simulink model "robot_3DoF_model"  (R2023a)
settings: Solver=FixedStepDiscrete  StartTime=0.0  StopTime=Inf  FixedStep=Ts_integration  RelTol=1e-3  EnableMultiTasking=on
model workspace (MAT data in the model file):
  Board = Simulink.Parameter
  Board.Value = [0.4  0.4; 0.2  0.6; 0  0.4]
  Board.DataType = 'double'
  Board.Complexity = 'real'
  Board.Dimensions = [3 2]
  BoardStiffness = Simulink.Parameter
  BoardStiffness.Value = [1000  0  0; 0  0  0; 0  0  0]
  BoardStiffness.DataType = 'auto'
  BoardStiffness.Complexity = 'real'
  BoardStiffness.Dimensions = [3 3]
  HC_KfD = Simulink.Parameter
  HC_KfD.Value = [0.1  0  0; 0  0  0; 0  0  0]
  HC_KfD.DataType = 'double'
  HC_KfD.Complexity = 'real'
  HC_KfD.Dimensions = [3 3]
  HC_KfI = Simulink.Parameter
  HC_KfI.Value = [1  0  0; 0  0  0; 0  0  0]
  HC_KfI.DataType = 'double'
  HC_KfI.Complexity = 'real'
  HC_KfI.Dimensions = [3 3]
  HC_KfP = Simulink.Parameter
  HC_KfP.Value = [0.05  0  0; 0  0  0; 0  0  0]
  HC_KfP.DataType = 'double'
  HC_KfP.Complexity = 'real'
  HC_KfP.Dimensions = [3 3]
  HC_KpD = Simulink.Parameter
  HC_KpD.Value = [15  0  0; 0  15  0; 0  0  20]
  HC_KpD.DataType = 'double'
  HC_KpD.Complexity = 'real'
  HC_KpD.Dimensions = [3 3]
  HC_KpI = Simulink.Parameter
  HC_KpI.Value = [0.5  0  0; 0  0.5  0; 0  0  10]
  HC_KpI.DataType = 'double'
  HC_KpI.Complexity = 'real'
  HC_KpI.Dimensions = [3 3]
  HC_KpP = Simulink.Parameter
  HC_KpP.Value = [25  0  0; 0  25  0; 0  0  600]
  HC_KpP.DataType = 'double'
  HC_KpP.Complexity = 'real'
  HC_KpP.Dimensions = [3 3]
  HC_Selection = Simulink.Parameter
  HC_Selection.Value = [0  0  0; 0  1  0; 0  0  1]
  HC_Selection.DataType = 'double'
  HC_Selection.Complexity = 'real'
  HC_Selection.Dimensions = [3 3]
  HC_tau0 = Simulink.Parameter
  HC_tau0.Value = [0; 0; 12.3985]
  HC_tau0.DataType = 'double'
  HC_tau0.Complexity = 'real'
  HC_tau0.Dimensions = [3 1]
  SM_gamma = Simulink.Parameter
  SM_gamma.Value = 0.001
  SM_gamma.DataType = 'auto'
  SM_gamma.Complexity = 'real'
  SM_gamma.Dimensions = [1 1]
  SM_lambda = Simulink.Parameter
  SM_lambda.Value = 2
  SM_lambda.DataType = 'auto'
  SM_lambda.Complexity = 'real'
  SM_lambda.Dimensions = [1 1]
  SM_rho = Simulink.Parameter
  SM_rho.Value = 10
  SM_rho.DataType = 'auto'
  SM_rho.Complexity = 'real'
  SM_rho.Dimensions = [1 1]
  SM_slidingGain = Simulink.Parameter
  SM_slidingGain.Value = [0  0  0; 0  0  0; 0  0  0]
  SM_slidingGain.DataType = 'auto'
  SM_slidingGain.Complexity = 'real'
  SM_slidingGain.Dimensions = [3 3]
  SM_widthInverse = Simulink.Parameter
  SM_widthInverse.Value = [100  0  0; 0  100  0; 0  0  100]
  SM_widthInverse.DataType = 'auto'
  SM_widthInverse.Complexity = 'real'
  SM_widthInverse.Dimensions = [3 3]
  Ts_control = Simulink.Parameter
  Ts_control.Value = 0.01
  Ts_control.DataType = 'double'
  Ts_control.Complexity = 'real'
  Ts_control.Dimensions = [1 1]
  Ts_integration = Simulink.Parameter
  Ts_integration.Value = 0.001
  Ts_integration.DataType = 'double'
  Ts_integration.Complexity = 'real'
  Ts_integration.Dimensions = [1 1]
  q_initial = Simulink.Parameter
  q_initial.Value = [2.00142; -1.6713; -0.21737; 0; 0; 0]
  q_initial.DataType = 'double'
  q_initial.Complexity = 'real'
  q_initial.Dimensions = [6 1]
  q_res1 = Simulink.Parameter
  q_res1.Value = 628318
  q_res1.DataType = 'auto'
  q_res1.Complexity = 'real'
  q_res1.Dimensions = [1 1]
  q_res2 = Simulink.Parameter
  q_res2.Value = 628318
  q_res2.DataType = 'auto'
  q_res2.Complexity = 'real'
  q_res2.Dimensions = [1 1]
  q_res3 = Simulink.Parameter
  q_res3.Value = 628318
  q_res3.DataType = 'auto'
  q_res3.Complexity = 'real'
  q_res3.Dimensions = [1 1]
libraries: dspinverses x1
settings Model: Creator=devans  LastModifiedBy=admin
settings SolverCC: AlgebraicLoopSolver=TrustRegion
settings DataIOCC: SaveFormat=Array  SignalLoggingSaveFormat=ModelDataLogs  SaveOutput=off  SaveTime=off  ReturnWorkspaceOutputs=off  SignalLoggingName=sigsOut
settings OptimizationCC: ExpressionDepthLimit=2147483647  LifeSpan=inf
settings DebuggingCC: SaveWithParameterizedLinksMsg=none  UnderspecifiedInitializationDetection=Classic  MergeDetectMultiDrivingBlocksExec=none  SignalResolutionControl=TryResolveAllWithWarning  MultiTaskDSMMsg=warning  MultiTaskCondExecSysMsg=none  UnconnectedInputMsg=warning  UnconnectedOutputMsg=warning  UnconnectedLineMsg=warning  StateNameClashWarn=warning  SFUnexpectedBacktrackingDiag=warning  SFNoUnconditionalDefaultTransitionDiag=warning  SFExecutionAtInitializationDiag=none  ArithmeticOperatorsInVariantConditions=warning
settings HardwareCC: ProdBitPerPointer=32  ProdBitPerSizeT=32  ProdBitPerPtrDiffT=32  ProdLargestAtomicFloat=None  ProdIntDivRoundTo=Undefined  ProdEndianess=Unspecified  ProdWordSize=32  ProdHWDeviceType=32-bit Generic  TargetBitPerPointer=64  TargetBitPerSizeT=64  TargetBitPerPtrDiffT=64  TargetLongLongMode=on  TargetIntDivRoundTo=Zero  TargetEndianess=LittleEndian  TargetWordSize=64  TargetHWDeviceType=MATLAB Host  ProdEqTarget=off
settings ModelReferenceCC: PropagateSignalLabelsOutOfModel=off
settings SFSimCC: SimUseLocalCustomCode=off  CustomCodeUndefinedFunction=UseInterfaceOnly
settings RTWCC: RTWUseLocalCustomCode=off
settings CodeAppCC: StateflowObjectComments=on
settings GRTTargetCC: TargetLangStandard=C89/C90 (ANSI)  CombineOutputUpdateFcns=off  GRTInterface=on
settings ConfigComp: CovMetricSettings=dw  CovSaveCumulativeToWorkspaceVar=on  CovSaveSingleToWorkspaceVar=on  CovExternalEMLEnable=off

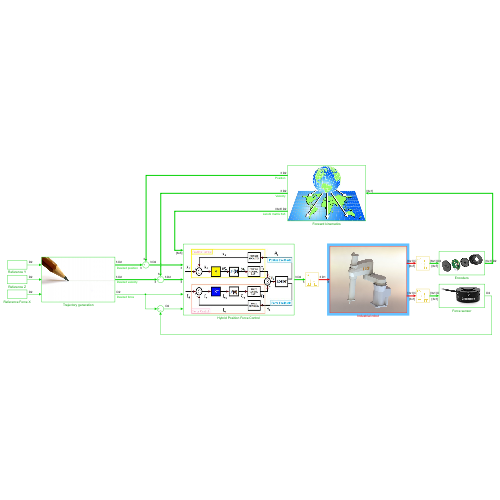
[thumbnail: Simulink's stored preview of the top-level diagram]
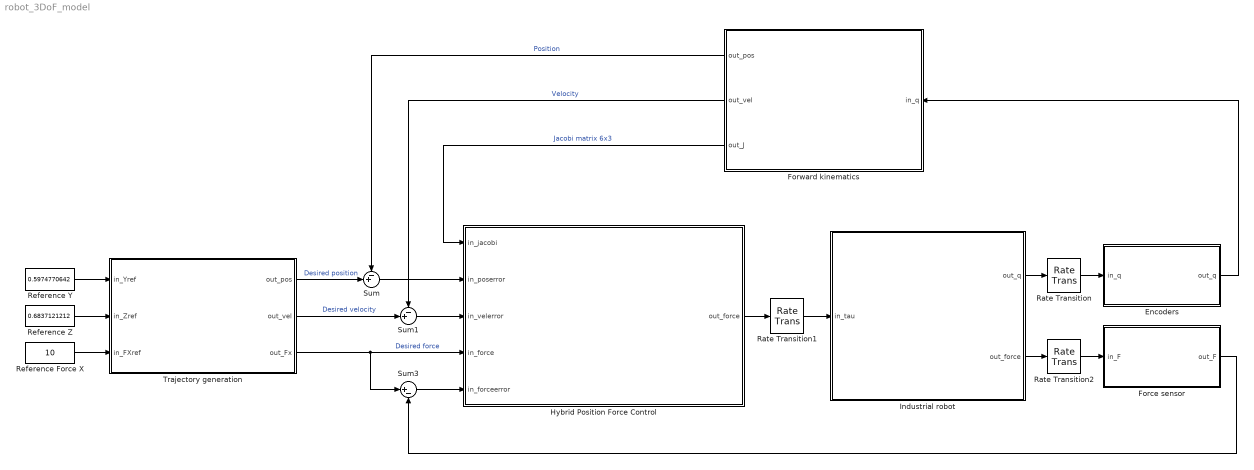
== system robot_3DoF_model ==
  Encoders : Subsystem
      mask Display: image('./Media/MR-Encoder.jpg');
  Force sensor : Subsystem
      mask Display: image('./Media/forcesensor.jpg');
  Forward kinematics : Subsystem
      mask Display: image('./Media/inverse.jpg');
  Hybrid Position Force Control : Subsystem
      mask Display: image('./Media/hybridcontrol.jpg');
  Industrial robot : Subsystem
      mask Display: image('./Media/3DoFrobot.jpg');
  Rate Transition : RateTransition  InitialCondition=q_initial  OutPortSampleTime=Ts_control
  Rate Transition1 : RateTransition  InitialCondition=[0;0;0]  OutPortSampleTime=Ts_integration
  Rate Transition2 : RateTransition  InitialCondition=[0;0;0]  OutPortSampleTime=Ts_control
  Reference Force X : Constant  Value=10  OutMin=5  OutMax=20  SampleTime=Ts_control
  Reference Y : Constant  Value=0.5974770642  OutMin=0  OutMax=1  SampleTime=Ts_control
  Reference Z : Constant  Value=0.6837121212  OutMin=0  OutMax=1  SampleTime=Ts_control
  Sum : Sum  Inputs=-+|
  Sum1 : Sum  Inputs=-+|
  Sum3 : Sum  Inputs=|+-
  Trajectory generation : Subsystem
      mask Display: image('./Media/draw-the-line.jpg');
  wires:
  Industrial robot/1(out_q) -> Rate Transition/1
  Rate Transition/1 -> Encoders/1(in_q)
  Encoders/1(out_q) -> Forward kinematics/1(in_q)
  Trajectory generation/1(out_pos) -> Sum/2  "Desired position"
  Forward kinematics/1(out_pos) -> Sum/1  "Position"
  Trajectory generation/2(out_vel) -> Sum1/2  "Desired velocity"
  Forward kinematics/2(out_vel) -> Sum1/1  "Velocity"
  Sum1/1 -> Hybrid Position Force Control/3(in_velerror)
  Forward kinematics/3(out_J) -> Hybrid Position Force Control/1(in_jacobi)  "Jacobi matrix 6x3"
  Rate Transition1/1 -> Industrial robot/1(in_tau)
  Hybrid Position Force Control/1(out_force) -> Rate Transition1/1
  Sum/1 -> Hybrid Position Force Control/2(in_poserror)
  Reference Y/1 -> Trajectory generation/1(in_Yref)
  Industrial robot/2(out_force) -> Rate Transition2/1
  Rate Transition2/1 -> Force sensor/1(in_F)
  Sum3/1 -> Hybrid Position Force Control/5(in_forceerror)
  Force sensor/1(out_F) -> Sum3/2
  Reference Z/1 -> Trajectory generation/2(in_Zref)
  Reference Force X/1 -> Trajectory generation/3(in_FXref)
  Trajectory generation/3(out_Fx) -> Hybrid Position Force Control/4(in_force), Sum3/1  "Desired force"

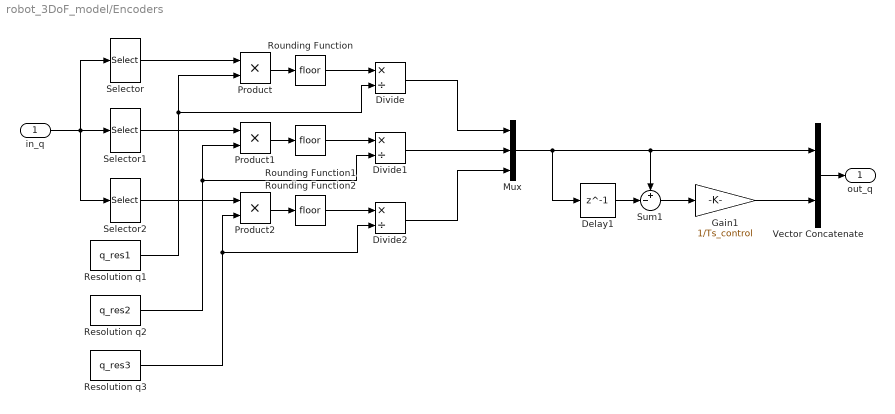
== system robot_3DoF_model/Encoders ==
  in_q : Inport
  Delay1 : Delay  DelayLength=1  InitialCondition=q_initial(1:3)
  Divide : Product  Inputs=*/
  Divide1 : Product  Inputs=*/
  Divide2 : Product  Inputs=*/
  Gain1 : Gain  Gain=1/Ts_control
  Mux : Mux  Inputs=3
  Product : Product  RndMeth=Zero
  Product1 : Product  RndMeth=Zero
  Product2 : Product  RndMeth=Zero
  Resolution q1 : Constant  Value=q_res1
  Resolution q2 : Constant  Value=q_res2
  Resolution q3 : Constant  Value=q_res3
  Rounding Function : Rounding
  Rounding Function1 : Rounding
  Rounding Function2 : Rounding
  Selector : Selector  InputPortWidth=6  IndexOptions=Index vector (dialog)  Indices=1  OutputSizes=1
  Selector1 : Selector  InputPortWidth=6  IndexOptions=Index vector (dialog)  Indices=2  OutputSizes=1
  Selector2 : Selector  InputPortWidth=6  IndexOptions=Index vector (dialog)  Indices=3  OutputSizes=1
  Sum1 : Sum  Inputs=+-|
  Vector Concatenate : Concatenate  Mode=Multidimensional array
  out_q : Outport
  wires:
  Product/1 -> Rounding Function/1
  Product1/1 -> Rounding Function1/1
  Product2/1 -> Rounding Function2/1
  Selector/1 -> Product/1
  Selector1/1 -> Product1/1
  Selector2/1 -> Product2/1
  Resolution q1/1 -> Product/2, Divide/2
  Resolution q2/1 -> Product1/2, Divide1/2
  Resolution q3/1 -> Divide2/2, Product2/2
  Rounding Function/1 -> Divide/1
  Rounding Function1/1 -> Divide1/1
  Rounding Function2/1 -> Divide2/1
  Divide/1 -> Mux/1
  Divide1/1 -> Mux/2
  Divide2/1 -> Mux/3
  in_q/1 -> Selector2/1, Selector1/1, Selector/1
  Mux/1 -> Delay1/1, Sum1/1, Vector Concatenate/1
  Delay1/1 -> Sum1/2
  Sum1/1 -> Gain1/1
  Gain1/1 -> Vector Concatenate/2
  Vector Concatenate/1 -> out_q/1

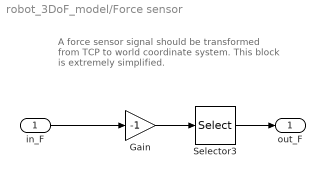
== system robot_3DoF_model/Force sensor ==
  note: A force sensor signal should be transformed
      | from TCP to world coordinate system.
      | This block is extremely simplified.
  in_F : Inport
  Gain : Gain  Gain=-1
  Selector3 : Selector  InputPortWidth=3  IndexOptions=Index vector (dialog)  Indices=1  OutputSizes=1
  out_F : Outport
  wires:
  in_F/1 -> Gain/1
  Gain/1 -> Selector3/1
  Selector3/1 -> out_F/1

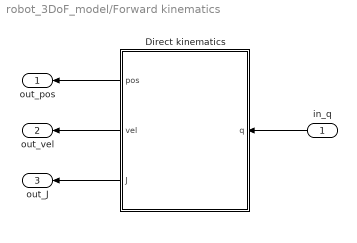
== system robot_3DoF_model/Forward kinematics ==
  in_q : Inport
  Direct kinematics : MATLAB Function  TreatAsAtomicUnit=on
  out_pos : Outport
  out_vel : Outport  Port=2
  out_J : Outport  Port=3
  wires:
  Direct kinematics/3(J) -> out_J/1
  in_q/1 -> Direct kinematics/1(q)
  Direct kinematics/2(vel) -> out_vel/1
  Direct kinematics/1(pos) -> out_pos/1

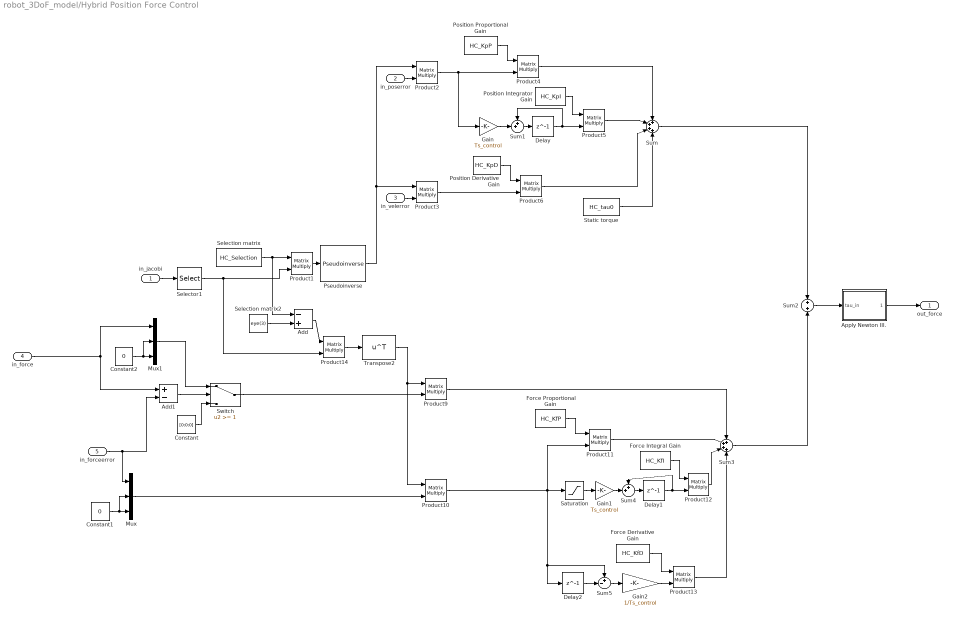
== system robot_3DoF_model/Hybrid Position Force Control ==
  in_jacobi : Inport
  in_poserror : Inport  Port=2
  in_velerror : Inport  Port=3
  in_force : Inport  Port=4
  in_forceerror : Inport  Port=5
  Add : Sum  Inputs=-+
  Add1 : Sum  Inputs=+-
  Apply Newton III. : MATLAB Function  TreatAsAtomicUnit=on
  Constant : Constant  Value=[0;0;0]
  Constant1 : Constant  Value=0
  Constant2 : Constant  Value=0
  Delay : Delay  DelayLength=1  InitialCondition=[0;0;0]
  Delay1 : Delay  DelayLength=1  InitialCondition=[0;0;0]
  Delay2 : Delay  DelayLength=1  InitialCondition=[0;0;0]
  Force Derivative Gain : Constant  Value=HC_KfD
  Force Integral Gain : Constant  Value=HC_KfI
  Force Proportional Gain : Constant  Value=HC_KfP
  Gain : Gain  Gain=Ts_control
  Gain1 : Gain  Gain=Ts_control
  Gain2 : Gain  Gain=1/Ts_control
  Mux : Mux  Inputs=3
  Mux1 : Mux  Inputs=3
  Position Derivative Gain : Constant  Value=HC_KpD
  Position Integrator Gain : Constant  Value=HC_KpI  VectorParams1D=off
  Position Proportional Gain : Constant  Value=HC_KpP
  Product{1..6,9..14} (12 alike) : Product  Multiplication=Matrix(*)  RndMeth=Zero
  Pseudoinverse : dspinverses/Pseudoinverse  wanterr=off  SimulateUsing=Interpreted execution
  Saturation : Saturate  UpperLimit=1  LowerLimit=-1
  Selection matrix : Constant  Value=HC_Selection
  Selection matrix2 : Constant  Value=eye(3)
  Selector1 : Selector  NumberOfDimensions=2  InputPortWidth=3  IndexOptions=Index vector (dialog),Index vector (dialog)  Indices=1:3,1:3  OutputSizes=1,1
  Static torque : Constant  Value=HC_tau0
  Sum : Sum  Inputs=++++
  Sum1 : Sum  Inputs=++|
  Sum2 : Sum
  Sum3 : Sum  Inputs=++++
  Sum4 : Sum  Inputs=++|
  Sum5 : Sum  Inputs=+-|
  Switch : Switch  Threshold=1  SaturateOnIntegerOverflow=off  InputSameDT=off
  Transpose2 : Math  Operator=transpose
  out_force : Outport
  wires:
  Product14/1 -> Transpose2/1
  Product2/1 -> Gain/1, Product4/2
  Position Proportional Gain/1 -> Product4/1
  Product4/1 -> Sum/1
  Sum1/1 -> Delay/1
  Delay/1 -> Product5/2, Sum1/1
  Gain/1 -> Sum1/2
  Position Integrator Gain/1 -> Product5/1
  Product5/1 -> Sum/2
  Position Derivative Gain/1 -> Product6/1
  Product3/1 -> Product6/2
  Product6/1 -> Sum/3
  Static torque/1 -> Sum/4
  Selection matrix/1 -> Add/1, Product1/1
  Add/1 -> Product14/1
  in_forceerror/1 -> Mux/1, Add1/2
  Sum/1 -> Sum2/1
  Sum3/1 -> Sum2/2
  Force Proportional Gain/1 -> Product11/1
  Saturation/1 -> Gain1/1
  Sum4/1 -> Delay1/1
  Gain1/1 -> Sum4/2
  Delay1/1 -> Product12/2, Sum4/1
  Force Integral Gain/1 -> Product12/1
  Product12/1 -> Sum3/3
  Product9/1 -> Sum3/1
  Add1/1 -> Switch/2
  Constant/1 -> Switch/3
  Product11/1 -> Sum3/2
  Product10/1 -> Delay2/1, Sum5/1, Product11/2, Saturation/1
  Delay2/1 -> Sum5/2
  Sum5/1 -> Gain2/1
  Gain2/1 -> Product13/2
  Force Derivative Gain/1 -> Product13/1
  Product13/1 -> Sum3/4
  Sum2/1 -> Apply Newton III./1(tau_in)
  Apply Newton III./1(tau_out) -> out_force/1
  Switch/1 -> Product9/2
  Transpose2/1 -> Product10/1, Product9/1
  Pseudoinverse/1 -> Product2/1, Product3/1
  Product1/1 -> Pseudoinverse/1
  Constant1/1 -> Mux/2, Mux/3
  in_velerror/1 -> Product3/2
  in_poserror/1 -> Product2/2
  in_jacobi/1 -> Selector1/1
  Mux1/1 -> Switch/1
  Constant2/1 -> Mux1/2, Mux1/3
  in_force/1 -> Mux1/1, Add1/1
  Selector1/1 -> Product1/2, Product14/2
  Mux/1 -> Product10/2
  Selection matrix2/1 -> Add/2

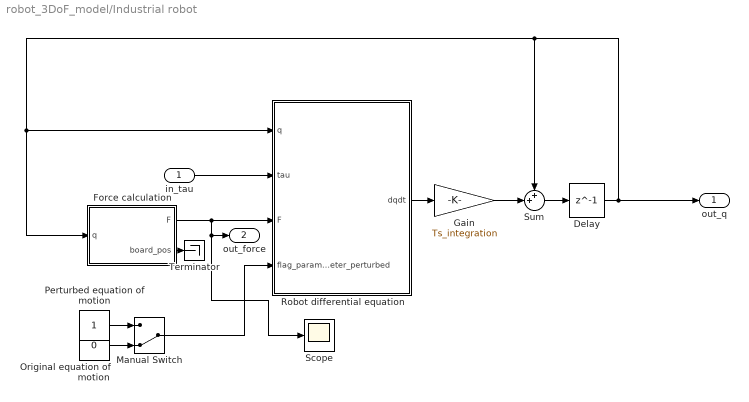
== system robot_3DoF_model/Industrial robot ==
  in_tau : Inport
  Delay : Delay  DelayLength=1  InitialCondition=q_initial
  Force calculation : MATLAB Function  TreatAsAtomicUnit=on
  Gain : Gain  Gain=Ts_integration
  Manual Switch : ManualSwitch  CurrentSetting=0
  Original equation of motion : Constant  Value=0
  Perturbed equation of motion : Constant
  Robot differential equation : MATLAB Function  TreatAsAtomicUnit=on
  Scope : Scope
  Sum : Sum  Inputs=++|
  Terminator : Terminator
  out_q : Outport
  out_force : Outport  Port=2
  wires:
  Robot differential equation/1(dqdt) -> Gain/1
  Gain/1 -> Sum/2
  Delay/1 -> out_q/1, Sum/1, Force calculation/1(q), Robot differential equation/1(q)
  Sum/1 -> Delay/1
  in_tau/1 -> Robot differential equation/2(tau)
  Force calculation/1(F) -> Robot differential equation/3(F), Scope/1, out_force/1
  Force calculation/2(board_pos) -> Terminator/1
  Perturbed equation of motion/1 -> Manual Switch/1
  Original equation of motion/1 -> Manual Switch/2
  Manual Switch/1 -> Robot differential equation/4(flag_parameter_perturbed)

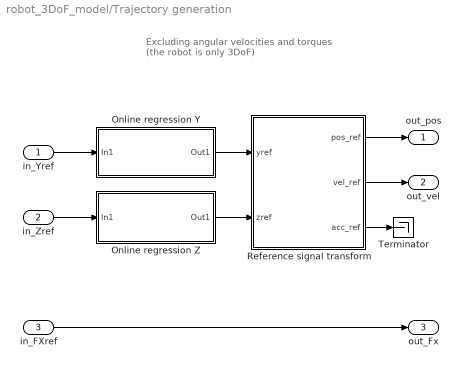
== system robot_3DoF_model/Trajectory generation ==
  note: Excluding angular velocities and torques
      | (the robot is only 3DoF)
  in_Yref : Inport
  in_Zref : Inport  Port=2
  in_FXref : Inport  Port=3
  Online regression Y : Subsystem  mask{d=2, lambda=0.99}
      mask prompts: d "Filter order"; lambda "Forgetfulness"
  Online regression Z : Subsystem  mask{d=2, lambda=0.99}
      mask prompts: d "Filter order"; lambda "Forgetfulness"
  Reference signal transform : MATLAB Function  TreatAsAtomicUnit=on
  Terminator : Terminator
  out_pos : Outport
  out_vel : Outport  Port=2
  out_Fx : Outport  Port=3
  wires:
  Reference signal transform/1(pos_ref) -> out_pos/1
  Reference signal transform/2(vel_ref) -> out_vel/1
  in_Yref/1 -> Online regression Y/1(In1)
  in_Zref/1 -> Online regression Z/1(In1)
  in_FXref/1 -> out_Fx/1
  Online regression Y/1(Out1) -> Reference signal transform/1(yref)
  Online regression Z/1(Out1) -> Reference signal transform/2(zref)
  Reference signal transform/3(acc_ref) -> Terminator/1

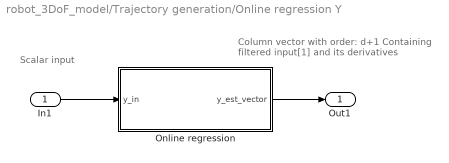
== system robot_3DoF_model/Trajectory generation/Online regression Y ==
  note: Column vector with order: d+1
      | Containing filtered input[1] and its derivatives
  note: Scalar input
  In1 : Inport
  Online regression : MATLAB Function  TreatAsAtomicUnit=on
  Out1 : Outport
  wires:
  In1/1 -> Online regression/1(y_in)
  Online regression/1(y_est_vector) -> Out1/1

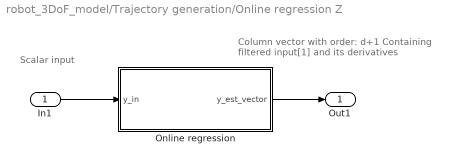
== system robot_3DoF_model/Trajectory generation/Online regression Z ==
  note: Scalar input
  note: Column vector with order: d+1
      | Containing filtered input[1] and its derivatives
  In1 : Inport
  Online regression : MATLAB Function  TreatAsAtomicUnit=on
  Out1 : Outport
  wires:
  Online regression/1(y_est_vector) -> Out1/1
  In1/1 -> Online regression/1(y_in)

== matlab function robot_3DoF_model/Industrial robot/Force calculation ==
  data: q input size=[6,1]; F output size=[3,1]; Board parameter; BoardStiffness parameter; board_pos output
function [F, board_pos]  = force(q, Board, BoardStiffness)
%#codegen

persistent XYZmin XYZrange
if isempty(XYZmin)
    XYZmin = min(Board,[],2);
    XYZrange = abs(Board([1,2,3],2)-Board([1,2,3],1));
end

q1 = q(1);
q2 = q(2);
q3 = q(3);
% qD1 = q(4);
% qD2 = q(5);
% qD3 = q(6);

pos = [0.25E0.*cos(q1)+0.52066E0.*cos(q1+q2)+0.114715E0.*sin(q1+q2);( ...
  -0.114715E0).*cos(q1+q2)+0.25E0.*sin(q1)+0.52066E0.*sin(q1+q2); ...
  0.41737E0+0.1E1.*q3];

disp = max([0;0;0],pos-XYZmin);

F = - BoardStiffness * disp;

% Relatív TCP helyzet 0...1 között
board_pos = (pos([2,3]) - XYZmin([2,3]))./ XYZrange([2,3]);

end

== matlab function robot_3DoF_model/Industrial robot/Robot differential equation ==
  data: q input size=[6,1]; tau input size=[3,1]; F input size=[3,1]; dqdt output; flag_parameter_perturbed input
function dqdt  = robot(q, tau, F, flag_parameter_perturbed)
%#codegen

persistent H_coef h_coef
if isempty(H_coef)
    H_coef = 0.6 + 0.8*rand(3,3);
    h_coef = 0.6 + 0.8*rand(3,1);
end

q1 = q(1);
q2 = q(2);
% q3 = q(3);
qD1 = q(4);
qD2 = q(5);
qD3 = q(6);

Fx = F(1);
Fy = F(2);
Fz = F(3);

tau1 = tau(1);
tau2 = tau(2);
tau3 = tau(3);

%   Apply Newton III.
tau = [tau1 - tau2;
        tau2;
        tau3];

q12 = q1 + q2;
S1 = sin(q1);
C1 = cos(q1);
S2 = sin(q2);
C2 = cos(q2);
S12 = sin(q12);
C12 = cos(q12);

H = [0.992754E0+0.611737E0.*C2+(-0.353817E-2).*S2, ...
  0.375243E0+0.305869E0.*C2+(-0.176909E-2).*S2,0; ...
  0.375243E0+0.305869E0.*C2+(-0.176909E-2).*S2,0.375243E0, ...
  0;0,0,0.126386E1];

h = [qD1.*qD2.*((-0.353817E-2).*C2+(-0.611737E0).*S2)+ ...
  qD2.^2.*((-0.176909E-2).*C2+(-0.305869E0).*S2);qD1.^2.*( ...
  0.176909E-2.*C2+0.305869E0.*S2);0.123985E2];

f = [Fx.*(0.114715E0.*C12+(-0.25E0).*S1+(-0.52066E0).*S12 ...
  )+Fy.*(0.25E0.*C1+0.52066E0.*C12+0.114715E0.* ...
  S12);Fx.*(0.114715E0.*C12+(-0.52066E0).*S12)+ ...
  Fy.*(0.52066E0.*C12+0.114715E0.*S12);0.1E1.*Fz];

if flag_parameter_perturbed > 0
    dqdt = cat(1,[qD1; qD2; qD3],...
        (H_coef.*H) \ (f + tau - h_coef.*h));
else
    dqdt = cat(1,[qD1; qD2; qD3],...
        H \ (f + tau - h));
end

end

== matlab function robot_3DoF_model/Forward kinematics/Direct kinematics ==
  data: q input; pos output; vel output; J output
function [pos, vel, J] = FwKin(q)
%#codegen

q1 = q(1);
q2 = q(2);
q3 = q(3);
qD1 = q(4);
qD2 = q(5);
qD3 = q(6);

pos = [0.25E0.*cos(q1)+0.52066E0.*cos(q1+q2)+0.114715E0.*sin(q1+q2);( ...
  -0.114715E0).*cos(q1+q2)+0.25E0.*sin(q1)+0.52066E0.*sin(q1+q2); ...
  0.41737E0+0.1E1.*q3];

Jv = [0.114715E0.*cos(q1+q2)+(-0.25E0).*sin(q1)+(-0.52066E0).*sin(q1+ ...
  q2),0.114715E0.*cos(q1+q2)+(-0.52066E0).*sin(q1+q2),0;0.25E0.*cos( ...
  q1)+0.52066E0.*cos(q1+q2)+0.114715E0.*sin(q1+q2),0.52066E0.*cos( ...
  q1+q2)+0.114715E0.*sin(q1+q2),0;0,0,0.1E1];

vel = Jv*[qD1;qD2;qD3];

Jom = [0,0,0;0,0,0;1.E0,1.E0,0];

J = cat(1,Jv,Jom);

end

== matlab function robot_3DoF_model/Trajectory generation/Reference signal transform ==
  data: yref input; pos_ref output; zref input; vel_ref output; Board parameter; acc_ref output
function [pos_ref, vel_ref, acc_ref] = ref_map(yref, zref, Board)
%#codegen

persistent XYZmin XYZrange
if isempty(XYZmin)
    XYZmin = min(Board,[],2);
    XYZrange = abs(Board([1,2,3],2)-Board([1,2,3],1));
end

pos_ref = XYZmin + XYZrange .* [0.4;yref(1);zref(1)];

vel_ref = XYZrange .* [0;yref(2);zref(2)];

acc_ref = XYZrange .* [0;yref(3);zref(3)];

end

== matlab function robot_3DoF_model/Hybrid Position Force Control/Apply Newton III. ==
  data: tau_out output; tau_in input
function tau_out = newtonIII(tau_in)
%#codegen

tau1 = tau_in(1);
tau2 = tau_in(2);
tau3 = tau_in(3);

tau_out = [tau1 + tau2;
            tau2;
            tau3];

end

== matlab function robot_3DoF_model/Trajectory generation/Online regression Y/Online regression ==
  data: y_est_vector output; y_in input size=1; Ts_control parameter size=1; d parameter size=1; lambda parameter size=1
function y_est_vector = online_reg(y_in , Ts_control, d, lambda)
%#codegen

% Ts - sample time, specify in main simulink workspace
% d  - filter order
% lambda - forgetfulness: must be within 0 and 1

% y_est_vector - column vector order d+1, 
% y_est_vector(1) - filtered input
% y_est_vector(i) - i-th derivative of filtered input up to order d

persistent L_i phi_0 P TH fact_mx
if isempty(L_i)
    
    % matrix for shifting measurements back with one step
    L = eye(d+1);
    for ii = 1:(d+1)
        for jj = 1:(d+1)
            if jj < ii
                L(ii,jj) = nchoosek(ii-1,jj-1) * (-Ts_control)^(ii-jj);
            end
        end
    end
    
    % inverse of a lower-triangular matrix
    L_i = eye(d+1);
    N = L - L_i;
    tmp = -N;
    for kk = 1:d
        L_i = L_i + tmp;
        tmp = tmp*(-N);
    end
    
    % creating factorial matrix for output
    fact_mx = diag(factorial(0:d));
    
    % initializing recursive variables
    phi_0 = [1;zeros(d,1)];
    P = eye(d+1);
    TH = zeros(d+1,1);
end

% K = L_i'*P*L_i;
% P = (eye(d+1) - K*(phi_0*phi_0') / (lambda + phi_0'*P*phi_0)) * K / lambda;
% L_iTH = L_i'*TH;
% TH = L_iTH + P*phi_0*(y_in - phi_0'*L_iTH);
% TH = TH + P*phi_0*(y_in - phi_0'*TH);

% y_est_vector = fact_mx * TH;

K = P*phi_0/(lambda + phi_0'*P*phi_0);
P = (eye(d+1) - K*phi_0')*P / lambda;
TH = TH + K*(y_in - phi_0'*TH);

y_est_vector = fact_mx * TH;

P = L_i'*P*L_i;
TH = L_i'*TH;

end

== matlab function robot_3DoF_model/Trajectory generation/Online regression Z/Online regression ==
  data: y_est_vector output; y_in input size=1; Ts_control parameter size=1; d parameter size=1; lambda parameter size=1
function y_est_vector = online_reg(y_in , Ts_control, d, lambda)
%#codegen

% Ts - sample time, specify in main simulink workspace
% d  - filter order
% lambda - forgetfulness: must be within 0 and 1

% y_est_vector - column vector order d+1, 
% y_est_vector(1) - filtered input
% y_est_vector(i) - i-th derivative of filtered input up to order d

persistent L_i phi_0 P TH fact_mx
if isempty(L_i)
    
    % matrix for shifting measurements back with one step
    L = eye(d+1);
    for ii = 1:(d+1)
        for jj = 1:(d+1)
            if jj < ii
                L(ii,jj) = nchoosek(ii-1,jj-1) * (-Ts_control)^(ii-jj);
            end
        end
    end
    
    % inverse of a lower-triangular matrix
    L_i = eye(d+1);
    N = L - L_i;
    tmp = -N;
    for kk = 1:d
        L_i = L_i + tmp;
        tmp = tmp*(-N);
    end
    
    % creating factorial matrix for output
    fact_mx = diag(factorial(0:d));
    
    % initializing recursive variables
    phi_0 = [1;zeros(d,1)];
    P = eye(d+1);
    TH = zeros(d+1,1);
end

% K = L_i'*P*L_i;
% P = (eye(d+1) - K*(phi_0*phi_0') / (lambda + phi_0'*P*phi_0)) * K / lambda;
% L_iTH = L_i'*TH;
% TH = L_iTH + P*phi_0*(y_in - phi_0'*L_iTH);
% TH = TH + P*phi_0*(y_in - phi_0'*TH);

% y_est_vector = fact_mx * TH;

K = P*phi_0/(lambda + phi_0'*P*phi_0);
P = (eye(d+1) - K*phi_0')*P / lambda;
TH = TH + K*(y_in - phi_0'*TH);

y_est_vector = fact_mx * TH;

P = L_i'*P*L_i;
TH = L_i'*TH;

end
